simulink model "CryoDetHcd"  (R2016b)
settings: Solver=ode45  StartTime=0.0  StopTime=1e-3  RelTol=1e-3
PreLoadFcn:
  | setup_hcd
values from neighbouring files (symbols this model uses):
  A = sqrt(0.5*erfc(x))    [setup_hcd.m]
  Fadc = 307.2e6    (= 307200000)    [setupADCtoDACloopback.m]    (also in setupCryoFPGA_CMB.m; setup_hcd.m = 614000000)
undefined symbols (not defined in the file or in its folder): AXI4, B, C, D, etaRomData, freqRomData, freqRomData1, freqRomData2, freqRomData3, j, Lite
libraries: xbsIndex_r4 x897, CryoDetLibCMB x8, hdlsllib x8, dspsigops x2, simulink x1
(part 6 of 8)

== system CryoDetHcd/DspCore/DSP/analysis_pipelined/Analysis0/channel_select1 ==
  tready : Inport
  data_valid : Inport  Port=2
  Constant : xbsIndex_r4/Constant  const=6  gui_display_data_type=Fixed-point  arith_type=Unsigned  n_bits=3  bin_pt=0  preci_type=Single  exp_width=8  frac_width=24  explicit_period=off  period=1  equ=P=C  opselect=C  inp2=PCIN>>17  opr=+  inp1=P  carry=CIN  dbl_ovrd=off  block_type=constant
  Counter : xbsIndex_r4/Counter  cnt_type=Free Running  cnt_to=Inf  operation=Up  start_count=0  cnt_by_val=1  arith_type=Unsigned  n_bits=3  bin_pt=0  load_pin=off  rst=on  en=on  explicit_period=on  period=2/Fadc  use_behavioral_HDL=off  implementation=Fabric  dbl_ovrd=off  block_type=counter
  Logical6 : xbsIndex_r4/Logical  logical_function=AND  inputs=2  en=off  latency=1  precision=Full  arith_type=Unsigned  n_bits=16  bin_pt=0  align_bp=on  dbl_ovrd=off  block_type=logical
  Relational : xbsIndex_r4/Relational  mode=a=b  op_type=Bool  en=off  latency=1  dbl_ovrd=off  block_type=relational
  tvalid : Outport
  tdata_fsel : Outport  Port=2
  t_last : Outport  Port=3
  wires:
  Logical6/1 -> Counter/2, tvalid/1
  data_valid/1 -> Logical6/2
  Counter/1 -> Relational/2, tdata_fsel/1
  tready/1 -> Logical6/1
  Relational/1 -> t_last/1
  Constant/1 -> Relational/1
  [reset] -> Counter/1

== system CryoDetHcd/DspCore/DSP/analysis_pipelined/Analysis0/scale1 ==
  note: do we saturate here or later???
  sel : Inport
  valid_i : Inport  Port=2
  In1 : Inport  Port=3
  Convert2 : xbsIndex_r4/Convert  gui_display_data_type=Boolean  arith_type=Boolean  n_bits=16  bin_pt=15  float_type=Single  exp_bits=8  fraction_bits=24  quantization=Truncate  overflow=Flag as error  en=off  latency=0  pipeline=off  dbl_ovrd=off  block_type=convert
  Delay : xbsIndex_r4/Delay  rst=off  infoeditControl=Selection of Reset will increase slice count due to use of real FFs and instead of SRLs  en=off  latency=1  reg_retiming=off  dbl_ovrd=off  block_type=delay
  Delay1 : xbsIndex_r4/Delay  rst=off  infoeditControl=Selection of Reset will increase slice count due to use of real FFs and instead of SRLs  en=off  latency=1  reg_retiming=off  dbl_ovrd=off  block_type=delay
  Delay2 : xbsIndex_r4/Delay  rst=off  infoeditControl=Selection of Reset will increase slice count due to use of real FFs and instead of SRLs  en=off  latency=1  reg_retiming=off  dbl_ovrd=off  block_type=delay
  Mux1 : xbsIndex_r4/Mux  inputs=2  en=off  latency=1  precision=User Defined  arith_type="Signed  (2's comp)"  n_bits=18  bin_pt=17  quantization=Truncate  overflow=Saturate  dbl_ovrd=off  block_type=mux
  Mux2 : xbsIndex_r4/Mux  inputs=2  en=off  latency=1  precision=User Defined  arith_type="Signed  (2's comp)"  n_bits=18  bin_pt=17  quantization=Truncate  overflow=Saturate  dbl_ovrd=off  block_type=mux
  high : xbsIndex_r4/BitBasher  bitexpr=|  display_expr=off  sr_1=im_out  arith_type1="Signed  (2's comp)"  bin_pt1=17  sr_2=re_out  arith_type2="Signed  (2's comp)"  bin_pt2=17  sr_3=indx  arith_type3=Unsigned  bin_pt3=0  sr_4=tlast  arith_type4=Unsigned  bin_pt4=0  dbl_ovrd=off  block_type=bitbasher
      | im_out ={ in[39:21] }
      | re_out = { in[18:0] }
      | indx    = { in[44:42] } 
      | tlast     = { in[45] }
  slice8 : xbsIndex_r4/BitBasher  bitexpr=|  display_expr=off  sr_1=im_out  arith_type1="Signed  (2's comp)"  bin_pt1=17  sr_2=re_out  arith_type2="Signed  (2's comp)"  bin_pt2=17  sr_3=indx  arith_type3=Unsigned  bin_pt3=0  sr_4=tlast  arith_type4=Unsigned  bin_pt4=0  dbl_ovrd=off  block_type=bitbasher
      | im_out ={ in[39:22] }
      | re_out = { in[18:1] }
      | indx    = { in[44:42] } 
      | tlast     = { in[45] }
  valid_o : Outport
  im : Outport  Port=2
  re : Outport  Port=3
  indx : Outport  Port=4
  tlast : Outport  Port=5
  wires:
  Convert2/1 -> Delay2/1
  In1/1 -> slice8/1, high/1
  high/3 -> Delay1/1
  high/4 -> Convert2/1
  high/2 -> Mux1/3
  slice8/2 -> Mux1/2
  Mux1/1 -> re/1
  high/1 -> Mux2/3
  Delay2/1 -> tlast/1
  valid_i/1 -> Delay/1
  slice8/1 -> Mux2/2
  Delay/1 -> valid_o/1
  Mux2/1 -> im/1
  Delay1/1 -> indx/1
  sel/1 -> Mux2/1, Mux1/1

== system CryoDetHcd/DspCore/DSP/analysis_pipelined/Analysis0/scale2 ==
  note: do we saturate here or later???
  sel : Inport
  valid_i : Inport  Port=2
  In1 : Inport  Port=3
  Delay : xbsIndex_r4/Delay  rst=off  infoeditControl=Selection of Reset will increase slice count due to use of real FFs and instead of SRLs  en=off  latency=1  reg_retiming=off  dbl_ovrd=off  block_type=delay
  Delay1 : xbsIndex_r4/Delay  rst=off  infoeditControl=Selection of Reset will increase slice count due to use of real FFs and instead of SRLs  en=off  latency=1  reg_retiming=off  dbl_ovrd=off  block_type=delay
  Mux1 : xbsIndex_r4/Mux  inputs=2  en=off  latency=1  precision=User Defined  arith_type="Signed  (2's comp)"  n_bits=18  bin_pt=17  quantization=Truncate  overflow=Saturate  dbl_ovrd=off  block_type=mux
  Mux2 : xbsIndex_r4/Mux  inputs=2  en=off  latency=1  precision=User Defined  arith_type="Signed  (2's comp)"  n_bits=18  bin_pt=17  quantization=Truncate  overflow=Saturate  dbl_ovrd=off  block_type=mux
  high : xbsIndex_r4/BitBasher  bitexpr=|  display_expr=off  sr_1=re  arith_type1="Signed  (2's comp)"  bin_pt1=17  sr_2=im  arith_type2="Signed  (2's comp)"  bin_pt2=17  sr_3=indx  arith_type3=Unsigned  bin_pt3=0  sr_4=4  arith_type4=Unsigned  bin_pt4=0  dbl_ovrd=off  block_type=bitbasher
      | re={in[18:0]}
      | im={in[44:26]}
      | indx ={in[54:52]}
  nominal : xbsIndex_r4/BitBasher  bitexpr=|  display_expr=off  sr_1=re  arith_type1="Signed  (2's comp)"  bin_pt1=17  sr_2=im  arith_type2="Signed  (2's comp)"  bin_pt2=17  sr_3=indx  arith_type3=Unsigned  bin_pt3=0  sr_4=4  arith_type4=Unsigned  bin_pt4=0  dbl_ovrd=off  block_type=bitbasher
      | re={in[18:1]}
      | im={in[44:27]}
      | indx ={in[54:52]}
  valid_o : Outport
  re : Outport  Port=2
  im : Outport  Port=3
  indx : Outport  Port=4
  wires:
  sel/1 -> Mux1/1, Mux2/1
  Delay1/1 -> indx/1
  Delay/1 -> valid_o/1
  valid_i/1 -> Delay/1
  In1/1 -> nominal/1, high/1
  Mux2/1 -> re/1
  Mux1/1 -> im/1
  high/3 -> Delay1/1
  high/2 -> Mux1/3
  high/1 -> Mux2/3
  nominal/1 -> Mux2/2
  nominal/2 -> Mux1/2

== system CryoDetHcd/DspCore/DSP/analysis_pipelined/Analysis0/scale3 ==
  note: do we saturate here or later???
  sel : Inport
  valid_i : Inport  Port=2
  In1 : Inport  Port=3
  Delay : xbsIndex_r4/Delay  rst=off  infoeditControl=Selection of Reset will increase slice count due to use of real FFs and instead of SRLs  en=off  latency=1  reg_retiming=off  dbl_ovrd=off  block_type=delay
  Delay1 : xbsIndex_r4/Delay  rst=off  infoeditControl=Selection of Reset will increase slice count due to use of real FFs and instead of SRLs  en=off  latency=1  reg_retiming=off  dbl_ovrd=off  block_type=delay
  Mux1 : xbsIndex_r4/Mux  inputs=2  en=off  latency=1  precision=User Defined  arith_type="Signed  (2's comp)"  n_bits=18  bin_pt=17  quantization=Truncate  overflow=Saturate  dbl_ovrd=off  block_type=mux
  Mux2 : xbsIndex_r4/Mux  inputs=2  en=off  latency=1  precision=User Defined  arith_type="Signed  (2's comp)"  n_bits=18  bin_pt=17  quantization=Truncate  overflow=Saturate  dbl_ovrd=off  block_type=mux
  high : xbsIndex_r4/BitBasher  bitexpr=|  display_expr=off  sr_1=re  arith_type1="Signed  (2's comp)"  bin_pt1=17  sr_2=im  arith_type2="Signed  (2's comp)"  bin_pt2=17  sr_3=indx  arith_type3=Unsigned  bin_pt3=0  sr_4=4  arith_type4=Unsigned  bin_pt4=0  dbl_ovrd=off  block_type=bitbasher
      | re={in[18:0]}
      | im={in[44:26]}
      | indx ={in[54:52]}
  nominal : xbsIndex_r4/BitBasher  bitexpr=|  display_expr=off  sr_1=re  arith_type1="Signed  (2's comp)"  bin_pt1=17  sr_2=im  arith_type2="Signed  (2's comp)"  bin_pt2=17  sr_3=indx  arith_type3=Unsigned  bin_pt3=0  sr_4=4  arith_type4=Unsigned  bin_pt4=0  dbl_ovrd=off  block_type=bitbasher
      | re={in[18:1]}
      | im={in[44:27]}
      | indx ={in[54:52]}
  valid_o : Outport
  re : Outport  Port=2
  im : Outport  Port=3
  indx : Outport  Port=4
  wires:
  nominal/2 -> Mux1/2
  nominal/1 -> Mux2/2
  high/1 -> Mux2/3
  high/2 -> Mux1/3
  high/3 -> Delay1/1
  Mux1/1 -> im/1
  Mux2/1 -> re/1
  In1/1 -> high/1, nominal/1
  valid_i/1 -> Delay/1
  Delay/1 -> valid_o/1
  Delay1/1 -> indx/1
  sel/1 -> Mux2/1, Mux1/1

== system CryoDetHcd/DspCore/DSP/analysis_pipelined/Analysis0/scale4 ==
  note: do we saturate here or later???
  sel : Inport
  valid_i : Inport  Port=2
  In1 : Inport  Port=3
  Convert2 : xbsIndex_r4/Convert  gui_display_data_type=Boolean  arith_type=Boolean  n_bits=16  bin_pt=15  float_type=Single  exp_bits=8  fraction_bits=24  quantization=Truncate  overflow=Flag as error  en=off  latency=0  pipeline=off  dbl_ovrd=off  block_type=convert
  Delay : xbsIndex_r4/Delay  rst=off  infoeditControl=Selection of Reset will increase slice count due to use of real FFs and instead of SRLs  en=off  latency=1  reg_retiming=off  dbl_ovrd=off  block_type=delay
  Delay1 : xbsIndex_r4/Delay  rst=off  infoeditControl=Selection of Reset will increase slice count due to use of real FFs and instead of SRLs  en=off  latency=1  reg_retiming=off  dbl_ovrd=off  block_type=delay
  Delay2 : xbsIndex_r4/Delay  rst=off  infoeditControl=Selection of Reset will increase slice count due to use of real FFs and instead of SRLs  en=off  latency=1  reg_retiming=off  dbl_ovrd=off  block_type=delay
  Mux1 : xbsIndex_r4/Mux  inputs=2  en=off  latency=1  precision=User Defined  arith_type="Signed  (2's comp)"  n_bits=18  bin_pt=17  quantization=Truncate  overflow=Saturate  dbl_ovrd=off  block_type=mux
  Mux2 : xbsIndex_r4/Mux  inputs=2  en=off  latency=1  precision=User Defined  arith_type="Signed  (2's comp)"  n_bits=18  bin_pt=17  quantization=Truncate  overflow=Saturate  dbl_ovrd=off  block_type=mux
  high : xbsIndex_r4/BitBasher  bitexpr=|  display_expr=off  sr_1=im_out  arith_type1="Signed  (2's comp)"  bin_pt1=17  sr_2=re_out  arith_type2="Signed  (2's comp)"  bin_pt2=17  sr_3=indx  arith_type3=Unsigned  bin_pt3=0  sr_4=tlast  arith_type4=Unsigned  bin_pt4=0  dbl_ovrd=off  block_type=bitbasher
      | im_out ={ in[39:21] }
      | re_out = { in[18:0] }
      | indx    = { in[44:42] } 
      | tlast     = { in[45] }
  slice8 : xbsIndex_r4/BitBasher  bitexpr=|  display_expr=off  sr_1=im_out  arith_type1="Signed  (2's comp)"  bin_pt1=17  sr_2=re_out  arith_type2="Signed  (2's comp)"  bin_pt2=17  sr_3=indx  arith_type3=Unsigned  bin_pt3=0  sr_4=tlast  arith_type4=Unsigned  bin_pt4=0  dbl_ovrd=off  block_type=bitbasher
      | im_out ={ in[39:22] }
      | re_out = { in[18:1] }
      | indx    = { in[44:42] } 
      | tlast     = { in[45] }
  valid_o : Outport
  im : Outport  Port=2
  re : Outport  Port=3
  indx : Outport  Port=4
  tlast : Outport  Port=5
  wires:
  sel/1 -> Mux1/1, Mux2/1
  Delay1/1 -> indx/1
  Mux2/1 -> im/1
  Delay/1 -> valid_o/1
  slice8/1 -> Mux2/2
  valid_i/1 -> Delay/1
  Delay2/1 -> tlast/1
  high/1 -> Mux2/3
  Mux1/1 -> re/1
  slice8/2 -> Mux1/2
  high/2 -> Mux1/3
  high/4 -> Convert2/1
  high/3 -> Delay1/1
  In1/1 -> high/1, slice8/1
  Convert2/1 -> Delay2/1

== system CryoDetHcd/DspCore/DSP/analysis_pipelined/Analysis1/channel_select1 ==
  tready : Inport
  data_valid : Inport  Port=2
  Constant : xbsIndex_r4/Constant  const=6  gui_display_data_type=Fixed-point  arith_type=Unsigned  n_bits=3  bin_pt=0  preci_type=Single  exp_width=8  frac_width=24  explicit_period=off  period=1  equ=P=C  opselect=C  inp2=PCIN>>17  opr=+  inp1=P  carry=CIN  dbl_ovrd=off  block_type=constant
  Counter : xbsIndex_r4/Counter  cnt_type=Free Running  cnt_to=Inf  operation=Up  start_count=0  cnt_by_val=1  arith_type=Unsigned  n_bits=3  bin_pt=0  load_pin=off  rst=on  en=on  explicit_period=on  period=2/Fadc  use_behavioral_HDL=off  implementation=Fabric  dbl_ovrd=off  block_type=counter
  Logical6 : xbsIndex_r4/Logical  logical_function=AND  inputs=2  en=off  latency=1  precision=Full  arith_type=Unsigned  n_bits=16  bin_pt=0  align_bp=on  dbl_ovrd=off  block_type=logical
  Relational : xbsIndex_r4/Relational  mode=a=b  op_type=Bool  en=off  latency=1  dbl_ovrd=off  block_type=relational
  tvalid : Outport
  tdata_fsel : Outport  Port=2
  t_last : Outport  Port=3
  wires:
  [reset] -> Counter/1
  Constant/1 -> Relational/1
  Relational/1 -> t_last/1
  tready/1 -> Logical6/1
  Counter/1 -> tdata_fsel/1, Relational/2
  data_valid/1 -> Logical6/2
  Logical6/1 -> tvalid/1, Counter/2

== system CryoDetHcd/DspCore/DSP/analysis_pipelined/Analysis1/scale1 ==
  note: do we saturate here or later???
  sel : Inport
  valid_i : Inport  Port=2
  In1 : Inport  Port=3
  Convert2 : xbsIndex_r4/Convert  gui_display_data_type=Boolean  arith_type=Boolean  n_bits=16  bin_pt=15  float_type=Single  exp_bits=8  fraction_bits=24  quantization=Truncate  overflow=Flag as error  en=off  latency=0  pipeline=off  dbl_ovrd=off  block_type=convert
  Delay : xbsIndex_r4/Delay  rst=off  infoeditControl=Selection of Reset will increase slice count due to use of real FFs and instead of SRLs  en=off  latency=1  reg_retiming=off  dbl_ovrd=off  block_type=delay
  Delay1 : xbsIndex_r4/Delay  rst=off  infoeditControl=Selection of Reset will increase slice count due to use of real FFs and instead of SRLs  en=off  latency=1  reg_retiming=off  dbl_ovrd=off  block_type=delay
  Delay2 : xbsIndex_r4/Delay  rst=off  infoeditControl=Selection of Reset will increase slice count due to use of real FFs and instead of SRLs  en=off  latency=1  reg_retiming=off  dbl_ovrd=off  block_type=delay
  Mux1 : xbsIndex_r4/Mux  inputs=2  en=off  latency=1  precision=User Defined  arith_type="Signed  (2's comp)"  n_bits=18  bin_pt=17  quantization=Truncate  overflow=Saturate  dbl_ovrd=off  block_type=mux
  Mux2 : xbsIndex_r4/Mux  inputs=2  en=off  latency=1  precision=User Defined  arith_type="Signed  (2's comp)"  n_bits=18  bin_pt=17  quantization=Truncate  overflow=Saturate  dbl_ovrd=off  block_type=mux
  high : xbsIndex_r4/BitBasher  bitexpr=|  display_expr=off  sr_1=im_out  arith_type1="Signed  (2's comp)"  bin_pt1=17  sr_2=re_out  arith_type2="Signed  (2's comp)"  bin_pt2=17  sr_3=indx  arith_type3=Unsigned  bin_pt3=0  sr_4=tlast  arith_type4=Unsigned  bin_pt4=0  dbl_ovrd=off  block_type=bitbasher
      | im_out ={ in[39:21] }
      | re_out = { in[18:0] }
      | indx    = { in[44:42] } 
      | tlast     = { in[45] }
  slice8 : xbsIndex_r4/BitBasher  bitexpr=|  display_expr=off  sr_1=im_out  arith_type1="Signed  (2's comp)"  bin_pt1=17  sr_2=re_out  arith_type2="Signed  (2's comp)"  bin_pt2=17  sr_3=indx  arith_type3=Unsigned  bin_pt3=0  sr_4=tlast  arith_type4=Unsigned  bin_pt4=0  dbl_ovrd=off  block_type=bitbasher
      | im_out ={ in[39:22] }
      | re_out = { in[18:1] }
      | indx    = { in[44:42] } 
      | tlast     = { in[45] }
  valid_o : Outport
  im : Outport  Port=2
  re : Outport  Port=3
  indx : Outport  Port=4
  tlast : Outport  Port=5
  wires:
  sel/1 -> Mux1/1, Mux2/1
  Delay1/1 -> indx/1
  Mux2/1 -> im/1
  Delay/1 -> valid_o/1
  slice8/1 -> Mux2/2
  valid_i/1 -> Delay/1
  Delay2/1 -> tlast/1
  high/1 -> Mux2/3
  Mux1/1 -> re/1
  slice8/2 -> Mux1/2
  high/2 -> Mux1/3
  high/4 -> Convert2/1
  high/3 -> Delay1/1
  In1/1 -> high/1, slice8/1
  Convert2/1 -> Delay2/1

== system CryoDetHcd/DspCore/DSP/analysis_pipelined/Analysis1/scale2 ==
  note: do we saturate here or later???
  sel : Inport
  valid_i : Inport  Port=2
  In1 : Inport  Port=3
  Delay : xbsIndex_r4/Delay  rst=off  infoeditControl=Selection of Reset will increase slice count due to use of real FFs and instead of SRLs  en=off  latency=1  reg_retiming=off  dbl_ovrd=off  block_type=delay
  Delay1 : xbsIndex_r4/Delay  rst=off  infoeditControl=Selection of Reset will increase slice count due to use of real FFs and instead of SRLs  en=off  latency=1  reg_retiming=off  dbl_ovrd=off  block_type=delay
  Mux1 : xbsIndex_r4/Mux  inputs=2  en=off  latency=1  precision=User Defined  arith_type="Signed  (2's comp)"  n_bits=18  bin_pt=17  quantization=Truncate  overflow=Saturate  dbl_ovrd=off  block_type=mux
  Mux2 : xbsIndex_r4/Mux  inputs=2  en=off  latency=1  precision=User Defined  arith_type="Signed  (2's comp)"  n_bits=18  bin_pt=17  quantization=Truncate  overflow=Saturate  dbl_ovrd=off  block_type=mux
  high : xbsIndex_r4/BitBasher  bitexpr=|  display_expr=off  sr_1=re  arith_type1="Signed  (2's comp)"  bin_pt1=17  sr_2=im  arith_type2="Signed  (2's comp)"  bin_pt2=17  sr_3=indx  arith_type3=Unsigned  bin_pt3=0  sr_4=4  arith_type4=Unsigned  bin_pt4=0  dbl_ovrd=off  block_type=bitbasher
      | re={in[18:0]}
      | im={in[44:26]}
      | indx ={in[54:52]}
  nominal : xbsIndex_r4/BitBasher  bitexpr=|  display_expr=off  sr_1=re  arith_type1="Signed  (2's comp)"  bin_pt1=17  sr_2=im  arith_type2="Signed  (2's comp)"  bin_pt2=17  sr_3=indx  arith_type3=Unsigned  bin_pt3=0  sr_4=4  arith_type4=Unsigned  bin_pt4=0  dbl_ovrd=off  block_type=bitbasher
      | re={in[18:1]}
      | im={in[44:27]}
      | indx ={in[54:52]}
  valid_o : Outport
  re : Outport  Port=2
  im : Outport  Port=3
  indx : Outport  Port=4
  wires:
  nominal/2 -> Mux1/2
  nominal/1 -> Mux2/2
  high/1 -> Mux2/3
  high/2 -> Mux1/3
  high/3 -> Delay1/1
  Mux1/1 -> im/1
  Mux2/1 -> re/1
  In1/1 -> high/1, nominal/1
  valid_i/1 -> Delay/1
  Delay/1 -> valid_o/1
  Delay1/1 -> indx/1
  sel/1 -> Mux2/1, Mux1/1

== system CryoDetHcd/DspCore/DSP/analysis_pipelined/Analysis1/scale3 ==
  note: do we saturate here or later???
  sel : Inport
  valid_i : Inport  Port=2
  In1 : Inport  Port=3
  Delay : xbsIndex_r4/Delay  rst=off  infoeditControl=Selection of Reset will increase slice count due to use of real FFs and instead of SRLs  en=off  latency=1  reg_retiming=off  dbl_ovrd=off  block_type=delay
  Delay1 : xbsIndex_r4/Delay  rst=off  infoeditControl=Selection of Reset will increase slice count due to use of real FFs and instead of SRLs  en=off  latency=1  reg_retiming=off  dbl_ovrd=off  block_type=delay
  Mux1 : xbsIndex_r4/Mux  inputs=2  en=off  latency=1  precision=User Defined  arith_type="Signed  (2's comp)"  n_bits=18  bin_pt=17  quantization=Truncate  overflow=Saturate  dbl_ovrd=off  block_type=mux
  Mux2 : xbsIndex_r4/Mux  inputs=2  en=off  latency=1  precision=User Defined  arith_type="Signed  (2's comp)"  n_bits=18  bin_pt=17  quantization=Truncate  overflow=Saturate  dbl_ovrd=off  block_type=mux
  high : xbsIndex_r4/BitBasher  bitexpr=|  display_expr=off  sr_1=re  arith_type1="Signed  (2's comp)"  bin_pt1=17  sr_2=im  arith_type2="Signed  (2's comp)"  bin_pt2=17  sr_3=indx  arith_type3=Unsigned  bin_pt3=0  sr_4=4  arith_type4=Unsigned  bin_pt4=0  dbl_ovrd=off  block_type=bitbasher
      | re={in[18:0]}
      | im={in[44:26]}
      | indx ={in[54:52]}
  nominal : xbsIndex_r4/BitBasher  bitexpr=|  display_expr=off  sr_1=re  arith_type1="Signed  (2's comp)"  bin_pt1=17  sr_2=im  arith_type2="Signed  (2's comp)"  bin_pt2=17  sr_3=indx  arith_type3=Unsigned  bin_pt3=0  sr_4=4  arith_type4=Unsigned  bin_pt4=0  dbl_ovrd=off  block_type=bitbasher
      | re={in[18:1]}
      | im={in[44:27]}
      | indx ={in[54:52]}
  valid_o : Outport
  re : Outport  Port=2
  im : Outport  Port=3
  indx : Outport  Port=4
  wires:
  sel/1 -> Mux1/1, Mux2/1
  Delay1/1 -> indx/1
  Delay/1 -> valid_o/1
  valid_i/1 -> Delay/1
  In1/1 -> nominal/1, high/1
  Mux2/1 -> re/1
  Mux1/1 -> im/1
  high/3 -> Delay1/1
  high/2 -> Mux1/3
  high/1 -> Mux2/3
  nominal/1 -> Mux2/2
  nominal/2 -> Mux1/2

== system CryoDetHcd/DspCore/DSP/analysis_pipelined/Analysis1/scale4 ==
  note: do we saturate here or later???
  sel : Inport
  valid_i : Inport  Port=2
  In1 : Inport  Port=3
  Convert2 : xbsIndex_r4/Convert  gui_display_data_type=Boolean  arith_type=Boolean  n_bits=16  bin_pt=15  float_type=Single  exp_bits=8  fraction_bits=24  quantization=Truncate  overflow=Flag as error  en=off  latency=0  pipeline=off  dbl_ovrd=off  block_type=convert
  Delay : xbsIndex_r4/Delay  rst=off  infoeditControl=Selection of Reset will increase slice count due to use of real FFs and instead of SRLs  en=off  latency=1  reg_retiming=off  dbl_ovrd=off  block_type=delay
  Delay1 : xbsIndex_r4/Delay  rst=off  infoeditControl=Selection of Reset will increase slice count due to use of real FFs and instead of SRLs  en=off  latency=1  reg_retiming=off  dbl_ovrd=off  block_type=delay
  Delay2 : xbsIndex_r4/Delay  rst=off  infoeditControl=Selection of Reset will increase slice count due to use of real FFs and instead of SRLs  en=off  latency=1  reg_retiming=off  dbl_ovrd=off  block_type=delay
  Mux1 : xbsIndex_r4/Mux  inputs=2  en=off  latency=1  precision=User Defined  arith_type="Signed  (2's comp)"  n_bits=18  bin_pt=17  quantization=Truncate  overflow=Saturate  dbl_ovrd=off  block_type=mux
  Mux2 : xbsIndex_r4/Mux  inputs=2  en=off  latency=1  precision=User Defined  arith_type="Signed  (2's comp)"  n_bits=18  bin_pt=17  quantization=Truncate  overflow=Saturate  dbl_ovrd=off  block_type=mux
  high : xbsIndex_r4/BitBasher  bitexpr=|  display_expr=off  sr_1=im_out  arith_type1="Signed  (2's comp)"  bin_pt1=17  sr_2=re_out  arith_type2="Signed  (2's comp)"  bin_pt2=17  sr_3=indx  arith_type3=Unsigned  bin_pt3=0  sr_4=tlast  arith_type4=Unsigned  bin_pt4=0  dbl_ovrd=off  block_type=bitbasher
      | im_out ={ in[39:21] }
      | re_out = { in[18:0] }
      | indx    = { in[44:42] } 
      | tlast     = { in[45] }
  slice8 : xbsIndex_r4/BitBasher  bitexpr=|  display_expr=off  sr_1=im_out  arith_type1="Signed  (2's comp)"  bin_pt1=17  sr_2=re_out  arith_type2="Signed  (2's comp)"  bin_pt2=17  sr_3=indx  arith_type3=Unsigned  bin_pt3=0  sr_4=tlast  arith_type4=Unsigned  bin_pt4=0  dbl_ovrd=off  block_type=bitbasher
      | im_out ={ in[39:22] }
      | re_out = { in[18:1] }
      | indx    = { in[44:42] } 
      | tlast     = { in[45] }
  valid_o : Outport
  im : Outport  Port=2
  re : Outport  Port=3
  indx : Outport  Port=4
  tlast : Outport  Port=5
  wires:
  Convert2/1 -> Delay2/1
  In1/1 -> slice8/1, high/1
  high/3 -> Delay1/1
  high/4 -> Convert2/1
  high/2 -> Mux1/3
  slice8/2 -> Mux1/2
  Mux1/1 -> re/1
  high/1 -> Mux2/3
  Delay2/1 -> tlast/1
  valid_i/1 -> Delay/1
  slice8/1 -> Mux2/2
  Delay/1 -> valid_o/1
  Mux2/1 -> im/1
  Delay1/1 -> indx/1
  sel/1 -> Mux2/1, Mux1/1

== system CryoDetHcd/DspCore/DSP/channel_processor/channel_processor_x1/Enabled Subsystem ==
  In1 : Inport
  In2 : Inport  Port=2
  Enable : EnablePort
  Buffer : Buffer  N=8  TreatMby1Signals=One channel  OutputFrames=off
  Buffer1 : Buffer  N=8  TreatMby1Signals=One channel  OutputFrames=off
  Out1 : Outport
  Out2 : Outport  Port=2
  wires:
  In1/1 -> Buffer/1
  Buffer/1 -> Out1/1
  In2/1 -> Buffer1/1
  Buffer1/1 -> Out2/1

== system CryoDetHcd/DspCore/DSP/channel_processor/channel_processor_x1/IQ_status_sel ==
  sel : Inport
  Q : Inport  Port=2
  I : Inport  Port=3
  ch : Inport  Port=4
  BitBasher : xbsIndex_r4/BitBasher  bitexpr=out = {I,Q}  display_expr=off  sr_1=out  arith_type1=Unsigned  bin_pt1=0  sr_2=2  arith_type2=Unsigned  bin_pt2=0  sr_3=3  arith_type3=Unsigned  bin_pt3=0  sr_4=4  arith_type4=Unsigned  bin_pt4=0  dbl_ovrd=off  block_type=bitbasher
  Convert : xbsIndex_r4/Convert  gui_display_data_type=Fixed-point  arith_type="Signed  (2's comp)"  n_bits=16  bin_pt=15  float_type=Single  exp_bits=8  fraction_bits=24  quantization=Truncate  overflow=Wrap  en=off  latency=1  pipeline=off  dbl_ovrd=off  block_type=convert
  Convert1 : xbsIndex_r4/Convert  gui_display_data_type=Fixed-point  arith_type="Signed  (2's comp)"  n_bits=16  bin_pt=15  float_type=Single  exp_bits=8  fraction_bits=24  quantization=Truncate  overflow=Wrap  en=off  latency=1  pipeline=off  dbl_ovrd=off  block_type=convert
  Register2 : xbsIndex_r4/Register  init=0  rst=off  en=on  dbl_ovrd=off  block_type=register
  Relational : xbsIndex_r4/Relational  mode=a=b  op_type=Bool  en=off  latency=1  dbl_ovrd=off  block_type=relational
  IQ_status_r : Outport
  wires:
  I/1 -> Convert1/1
  Q/1 -> Convert/1
  Convert1/1 -> BitBasher/2
  ch/1 -> Relational/2
  sel/1 -> Relational/1
  Convert/1 -> BitBasher/1
  BitBasher/1 -> Register2/1
  Register2/1 -> IQ_status_r/1
  Relational/1 -> Register2/2

== system CryoDetHcd/DspCore/DSP/channel_processor/channel_processor_x1/config2_r ==
  In1 : Inport
  BitBasher : xbsIndex_r4/BitBasher  bitexpr=|  display_expr=off  sr_1=ref_delay  arith_type1=Unsigned  bin_pt1=0  sr_2=tone_scale_sel  arith_type2=Unsigned  bin_pt2=0  sr_3=fb_enable  arith_type3=Unsigned  bin_pt3=0  sr_4=fb_polarity  arith_type4=Unsigned  bin_pt4=0  dbl_ovrd=off  block_type=bitbasher
      | ref_delay = {in[2:0]}
      | tone_scale_sel = {in[4:3]}
      | fb_enable = {in[5]}
      | fb_polarity = {in[6]}
  BitBasher1 : xbsIndex_r4/BitBasher  bitexpr=|  display_expr=off  sr_1=iq_swap_sel  arith_type1=Unsigned  bin_pt1=0  sr_2=iq_band_sel  arith_type2=Unsigned  bin_pt2=0  sr_3=iq_ch_sel  arith_type3=Unsigned  bin_pt3=0  sr_4=analysis_iq_ch_sel  arith_type4=Unsigned  bin_pt4=0  dbl_ovrd=off  block_type=bitbasher
      | iq_swap_sel = {in[7]}
      | iq_band_sel = {in[16:15]}
      | iq_ch_sel = {in[14:8]}
      | analysis_iq_ch_sel={in[17:15]}
  ref_delay : Outport
  tone_scale_sel : Outport  Port=2
  fb_enable : Outport  Port=3
  fb_polarity : Outport  Port=4
  iq_swap_sel : Outport  Port=5
  iq_band_sel : Outport  Port=6
  iq_ch_sel : Outport  Port=7
  analysis_iq_sel : Outport  Port=8
  wires:
  BitBasher1/3 -> iq_ch_sel/1
  BitBasher1/2 -> iq_band_sel/1
  BitBasher1/1 -> iq_swap_sel/1
  BitBasher/4 -> fb_polarity/1
  BitBasher/3 -> fb_enable/1
  BitBasher/2 -> tone_scale_sel/1
  BitBasher/1 -> ref_delay/1
  In1/1 -> BitBasher/1, BitBasher1/1
  BitBasher1/4 -> analysis_iq_sel/1

== system CryoDetHcd/DspCore/DSP/channel_processor/channel_processor_x1/config3_r1 ==
  In1 : Inport
  BitBasher1 : xbsIndex_r4/BitBasher  bitexpr=|  display_expr=off  sr_1=fb_gain  arith_type1=Unsigned  bin_pt1=14  sr_2=fb_limit  arith_type2=Unsigned  bin_pt2=16  sr_3=ref_delay  arith_type3=Unsigned  bin_pt3=0  sr_4=4  arith_type4=Unsigned  bin_pt4=0  dbl_ovrd=off  block_type=bitbasher
      | fb_gain = {in[15:0]}
      | fb_limit = {in[31:16]}
  Negate : xbsIndex_r4/Negate  precision=User Defined  arith_type=Unsigned  n_bits=16  bin_pt=15  quantization=Truncate  overflow=Wrap  en=off  latency=2  dbl_ovrd=off  block_type=negate
  fb_gain : Outport
  fb_limit_hi : Outport  Port=2
  fb_limit_lo : Outport  Port=3
  wires:
  BitBasher1/2 -> Negate/1, fb_limit_hi/1
  In1/1 -> BitBasher1/1
  BitBasher1/1 -> fb_gain/1
  Negate/1 -> fb_limit_lo/1

== system CryoDetHcd/DspCore/DSP/channel_processor/channel_processor_x1/scale1 ==
  In1 : Inport
  Bit Slice : hdlsllib/HDL Operations/Bit Slice  lidx=15  ridx=0
  Bit Slice1 : hdlsllib/HDL Operations/Bit Slice  lidx=31  ridx=16
  Data Type Conversion : DataTypeConversion  OutDataTypeStr=int16  ConvertRealWorld=Stored Integer (SI)
  Data Type Conversion1 : DataTypeConversion  OutDataTypeStr=int16  ConvertRealWorld=Stored Integer (SI)
  Q : Outport
  I : Outport  Port=2
  wires:
  In1/1 -> Bit Slice1/1, Bit Slice/1
  Bit Slice/1 -> Data Type Conversion/1
  Data Type Conversion1/1 -> Q/1
  Bit Slice1/1 -> Data Type Conversion1/1
  Data Type Conversion/1 -> I/1

== system CryoDetHcd/DspCore/DSP/channel_processor/channel_processor_x4/Enabled Subsystem ==
  In1 : Inport
  In2 : Inport  Port=2
  Enable : EnablePort
  Buffer : Buffer  N=8  TreatMby1Signals=One channel  OutputFrames=off
  Buffer1 : Buffer  N=8  TreatMby1Signals=One channel  OutputFrames=off
  Out1 : Outport
  Out2 : Outport  Port=2
  wires:
  In1/1 -> Buffer/1
  Buffer/1 -> Out1/1
  In2/1 -> Buffer1/1
  Buffer1/1 -> Out2/1

== system CryoDetHcd/DspCore/DSP/channel_processor/channel_processor_x4/config3_r ==
  In1 : Inport
  BitBasher1 : xbsIndex_r4/BitBasher  bitexpr=|  display_expr=off  sr_1=fb_gain  arith_type1=Unsigned  bin_pt1=14  sr_2=fb_limit  arith_type2=Unsigned  bin_pt2=16  sr_3=ref_delay  arith_type3=Unsigned  bin_pt3=0  sr_4=4  arith_type4=Unsigned  bin_pt4=0  dbl_ovrd=off  block_type=bitbasher
      | fb_gain = {in[15:0]}
      | fb_limit = {in[31:16]}
  Negate : xbsIndex_r4/Negate  precision=User Defined  arith_type=Unsigned  n_bits=16  bin_pt=15  quantization=Truncate  overflow=Wrap  en=off  latency=2  dbl_ovrd=off  block_type=negate
  fb_gain : Outport
  fb_limit_hi : Outport  Port=2
  fb_limit_lo : Outport  Port=3
  wires:
  BitBasher1/2 -> Negate/1, fb_limit_hi/1
  In1/1 -> BitBasher1/1
  BitBasher1/1 -> fb_gain/1
  Negate/1 -> fb_limit_lo/1

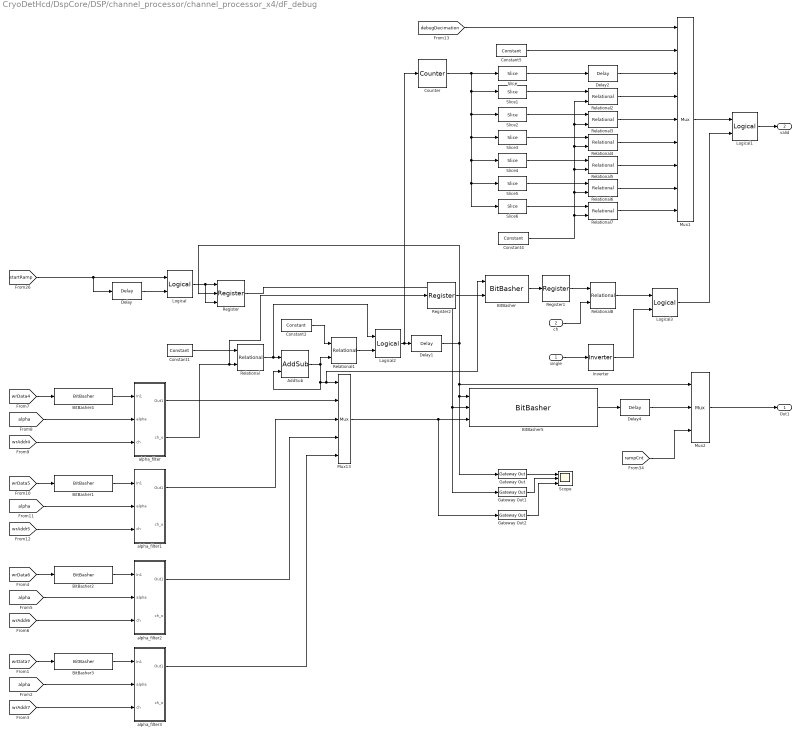
== system CryoDetHcd/DspCore/DSP/channel_processor/channel_processor_x4/dF_debug ==
  single : Inport
  ch : Inport  Port=2
  AddSub : xbsIndex_r4/AddSub  mode=Addition  use_carryin=off  use_carryout=off  en=off  latency=1  precision=User Defined  arith_type=Unsigned  n_bits=2  bin_pt=0  quantization=Truncate  overflow=Wrap  use_behavioral_HDL=off  hw_selection=Fabric  pipelined=off  dbl_ovrd=off  block_type=addsub
  BitBasher : xbsIndex_r4/BitBasher  bitexpr=out = {hi,lo}  display_expr=off  sr_1=out  arith_type1=Unsigned  bin_pt1=0  sr_2=channel_select  arith_type2=Unsigned  bin_pt2=0  sr_3=3  arith_type3=Unsigned  bin_pt3=0  sr_4=4  arith_type4=Unsigned  bin_pt4=0  dbl_ovrd=off  block_type=bitbasher
  BitBasher{1..4} (4 alike) : xbsIndex_r4/BitBasher  bitexpr=freq = {in[23:0]}  display_expr=on  sr_1=freq  arith_type1="Signed  (2's comp)"  bin_pt1=0  sr_2=2  arith_type2=Unsigned  bin_pt2=0  sr_3=3  arith_type3=Unsigned  bin_pt3=0  sr_4=4  arith_type4=Unsigned  bin_pt4=0  dbl_ovrd=off  block_type=bitbasher
  BitBasher5 : xbsIndex_r4/BitBasher  bitexpr=out = {flux_ramp, ch, 6'b0, freq}  display_expr=on  sr_1=out  arith_type1=Unsigned  bin_pt1=0  sr_2=2  arith_type2=Unsigned  bin_pt2=0  sr_3=3  arith_type3=Unsigned  bin_pt3=0  sr_4=4  arith_type4=Unsigned  bin_pt4=0  dbl_ovrd=off  block_type=bitbasher
  Constant1 : xbsIndex_r4/Constant  const=127  gui_display_data_type=Fixed-point  arith_type=Unsigned  n_bits=7  bin_pt=0  preci_type=Single  exp_width=8  frac_width=24  explicit_period=off  period=1  equ=P=C  opselect=C  inp2=PCIN>>17  opr=+  inp1=P  carry=CIN  dbl_ovrd=off  block_type=constant
  Constant2 : xbsIndex_r4/Constant  const=3  gui_display_data_type=Fixed-point  arith_type=Unsigned  n_bits=2  bin_pt=0  preci_type=Single  exp_width=8  frac_width=24  explicit_period=off  period=1  equ=P=C  opselect=C  inp2=PCIN>>17  opr=+  inp1=P  carry=CIN  dbl_ovrd=off  block_type=constant
  Constant4 : xbsIndex_r4/Constant  const=0  gui_display_data_type=Fixed-point  arith_type=Unsigned  n_bits=1  bin_pt=0  preci_type=Single  exp_width=8  frac_width=24  explicit_period=off  period=1  equ=P=C  opselect=C  inp2=PCIN>>17  opr=+  inp1=P  carry=CIN  dbl_ovrd=off  block_type=constant
  Constant5 : xbsIndex_r4/Constant  const=1  gui_display_data_type=Fixed-point  arith_type=Unsigned  n_bits=1  bin_pt=0  preci_type=Single  exp_width=8  frac_width=24  explicit_period=off  period=1  equ=P=C  opselect=C  inp2=PCIN>>17  opr=+  inp1=P  carry=CIN  dbl_ovrd=off  block_type=constant
  Counter : xbsIndex_r4/Counter  cnt_type=Free Running  cnt_to=Inf  operation=Up  start_count=0  cnt_by_val=1  arith_type=Unsigned  n_bits=7  bin_pt=0  load_pin=off  rst=off  en=on  explicit_period=off  period=2/Fadc  use_behavioral_HDL=off  implementation=Fabric  dbl_ovrd=off  block_type=counter
  Delay{,1..2,4} (4 alike) : xbsIndex_r4/Delay  rst=off  infoeditControl=Selection of Reset will increase slice count due to use of real FFs and instead of SRLs  en=off  latency=1  reg_retiming=off  dbl_ovrd=off  block_type=delay
  Gateway Out : xbsIndex_r4/Gateway Out  inherit_from_input=off  hdl_port=off  rows=1  columns=1  UseAsDAC=off  DACChannel='1'  interface=None  automatic_assignment=on  address_offset=hex2dec('00')  intf_name=''  intf_description=''  timing_constraint=None  locs_specified=off  LOCs={}  io_standard={}  block_type=gatewayout
  Gateway Out1 : xbsIndex_r4/Gateway Out  inherit_from_input=off  hdl_port=off  rows=1  columns=1  UseAsDAC=off  DACChannel='1'  interface=None  automatic_assignment=on  address_offset=hex2dec('00')  intf_name=''  intf_description=''  timing_constraint=None  locs_specified=off  LOCs={}  io_standard={}  block_type=gatewayout
  Gateway Out2 : xbsIndex_r4/Gateway Out  inherit_from_input=off  hdl_port=off  rows=1  columns=1  UseAsDAC=off  DACChannel='1'  interface=None  automatic_assignment=on  address_offset=hex2dec('00')  intf_name=''  intf_description=''  timing_constraint=None  locs_specified=off  LOCs={}  io_standard={}  block_type=gatewayout
  Inverter : xbsIndex_r4/Inverter  en=off  latency=0  dbl_ovrd=off  block_type=inv
  Logical : xbsIndex_r4/Logical  logical_function=OR  inputs=2  en=off  latency=1  precision=User Defined  arith_type=Boolean  n_bits=16  bin_pt=0  align_bp=on  dbl_ovrd=off  block_type=logical
  Logical1 : xbsIndex_r4/Logical  logical_function=AND  inputs=2  en=off  latency=0  precision=Full  arith_type=Unsigned  n_bits=16  bin_pt=0  align_bp=on  dbl_ovrd=off  block_type=logical
  Logical2 : xbsIndex_r4/Logical  logical_function=AND  inputs=2  en=off  latency=1  precision=User Defined  arith_type=Boolean  n_bits=16  bin_pt=0  align_bp=on  dbl_ovrd=off  block_type=logical
  Logical3 : xbsIndex_r4/Logical  logical_function=OR  inputs=2  en=off  latency=1  precision=Full  arith_type=Unsigned  n_bits=16  bin_pt=0  align_bp=on  dbl_ovrd=off  block_type=logical
  Mux1 : xbsIndex_r4/Mux  inputs=8  en=off  latency=1  precision=Full  arith_type=Unsigned  n_bits=16  bin_pt=14  quantization=Truncate  overflow=Wrap  dbl_ovrd=off  block_type=mux
  Mux13 : xbsIndex_r4/Mux  inputs=4  en=off  latency=1  precision=Full  arith_type=Unsigned  n_bits=16  bin_pt=14  quantization=Truncate  overflow=Wrap  dbl_ovrd=off  block_type=mux
  Mux2 : xbsIndex_r4/Mux  inputs=2  en=off  latency=1  precision=Full  arith_type=Unsigned  n_bits=16  bin_pt=14  quantization=Truncate  overflow=Wrap  dbl_ovrd=off  block_type=mux
  Register : xbsIndex_r4/Register  init=0  rst=on  en=on  dbl_ovrd=off  block_type=register
  Register1 : xbsIndex_r4/Register  init=0  rst=off  en=off  dbl_ovrd=off  block_type=register
  Register2 : xbsIndex_r4/Register  init=0  rst=off  en=off  dbl_ovrd=off  block_type=register
  Relational{,1..8} (9 alike) : xbsIndex_r4/Relational  mode=a=b  op_type=Ufix  en=off  latency=1  dbl_ovrd=off  block_type=relational
  Scope : Scope  NumInputPorts=3
  Slice : xbsIndex_r4/Slice  nbits=1  boolean_output=off  mode=Lower Bit Location + Width  bit1=0  base1=MSB of Input  bit0=0  base0=LSB of Input  dbl_ovrd=off  block_type=slice
  Slice1 : xbsIndex_r4/Slice  nbits=2  boolean_output=off  mode=Lower Bit Location + Width  bit1=0  base1=MSB of Input  bit0=0  base0=LSB of Input  dbl_ovrd=off  block_type=slice
  Slice2 : xbsIndex_r4/Slice  nbits=3  boolean_output=off  mode=Lower Bit Location + Width  bit1=0  base1=MSB of Input  bit0=0  base0=LSB of Input  dbl_ovrd=off  block_type=slice
  Slice3 : xbsIndex_r4/Slice  nbits=4  boolean_output=off  mode=Lower Bit Location + Width  bit1=0  base1=MSB of Input  bit0=0  base0=LSB of Input  dbl_ovrd=off  block_type=slice
  Slice4 : xbsIndex_r4/Slice  nbits=5  boolean_output=off  mode=Lower Bit Location + Width  bit1=0  base1=MSB of Input  bit0=0  base0=LSB of Input  dbl_ovrd=off  block_type=slice
  Slice5 : xbsIndex_r4/Slice  nbits=6  boolean_output=off  mode=Lower Bit Location + Width  bit1=0  base1=MSB of Input  bit0=0  base0=LSB of Input  dbl_ovrd=off  block_type=slice
  Slice6 : xbsIndex_r4/Slice  nbits=7  boolean_output=off  mode=Lower Bit Location + Width  bit1=0  base1=MSB of Input  bit0=0  base0=LSB of Input  dbl_ovrd=off  block_type=slice
  alpha_filter : Subsystem
  alpha_filter1 : Subsystem
  alpha_filter2 : Subsystem
  alpha_filter3 : Subsystem
  Out1 : Outport
  valid : Outport  Port=2
  wires:
  [wrData5] -> BitBasher1/1
  [alpha] -> alpha_filter1/2(alpha)
  [wrAddr4] -> alpha_filter/3(ch)
  [wrAddr5] -> alpha_filter1/3(ch)
  BitBasher1/1 -> alpha_filter1/1(In1)
  [alpha] -> alpha_filter/2(alpha)
  [wrData4] -> BitBasher4/1
  BitBasher4/1 -> alpha_filter/1(In1)
  [wrData7] -> BitBasher3/1
  [alpha] -> alpha_filter3/2(alpha)
  [wrAddr6] -> alpha_filter2/3(ch)
  [wrAddr7] -> alpha_filter3/3(ch)
  BitBasher3/1 -> alpha_filter3/1(In1)
  [alpha] -> alpha_filter2/2(alpha)
  [wrData6] -> BitBasher2/1
  BitBasher2/1 -> alpha_filter2/1(In1)
  alpha_filter/1(Out1) -> Mux13/2
  alpha_filter1/1(Out1) -> Mux13/3
  alpha_filter2/1(Out1) -> Mux13/4
  alpha_filter3/1(Out1) -> Mux13/5
  Delay/1 -> Logical/2
  [startRamp] -> Delay/1, Logical/1
  Logical/1 -> Register/3, Register/1
  alpha_filter/2(ch_o) -> Register2/1, Relational/2
  Constant1/1 -> Relational/1
  Constant2/1 -> Relational1/1
  Mux13/1 -> Gateway Out2/1, BitBasher5/3
  Relational1/1 -> Logical2/2
  Register/1 -> Gateway Out1/1, BitBasher5/2
  Relational/1 -> Logical2/1, AddSub/1
  Gateway Out/1 -> Scope/1
  Gateway Out1/1 -> Scope/2
  Gateway Out2/1 -> Scope/3
  Counter/1 -> Slice3/1, Slice4/1, Slice5/1, Slice6/1, Slice2/1, Slice1/1, Slice/1
  Logical2/1 -> Counter/1, Delay1/1
  Slice1/1 -> Relational2/1
  Slice2/1 -> Relational3/1
  Constant4/1 -> Relational2/2, Relational3/2, Relational4/2, Relational5/2, Relational6/2, Relational7/2
  Relational6/1 -> Mux1/8
  Relational5/1 -> Mux1/7
  Relational4/1 -> Mux1/6
  Relational3/1 -> Mux1/5
  Relational2/1 -> Mux1/4
  Delay2/1 -> Mux1/3
  Slice/1 -> Delay2/1
  Slice3/1 -> Relational4/1
  Slice4/1 -> Relational5/1
  Slice5/1 -> Relational6/1
  Slice6/1 -> Relational7/1
  Constant5/1 -> Mux1/2
  Relational7/1 -> Mux1/9
  Delay1/1 -> Register/2, Mux2/1, Gateway Out/1, BitBasher5/1
  Delay4/1 -> Mux2/2
  [rampCnt] -> Mux2/3
  BitBasher5/1 -> Delay4/1
  Mux2/1 -> Out1/1
  AddSub/1 -> AddSub/2, BitBasher/1, Mux13/1, Relational1/2
  BitBasher/1 -> Register1/1
  Register2/1 -> BitBasher/2
  Register1/1 -> Relational8/1
  Relational8/1 -> Logical3/1
  Logical3/1 -> Logical1/2
  ch/1 -> Relational8/2
  single/1 -> Inverter/1
  Inverter/1 -> Logical3/2
  Mux1/1 -> Logical1/1
  Logical1/1 -> valid/1
  [debugDecimation] -> Mux1/1

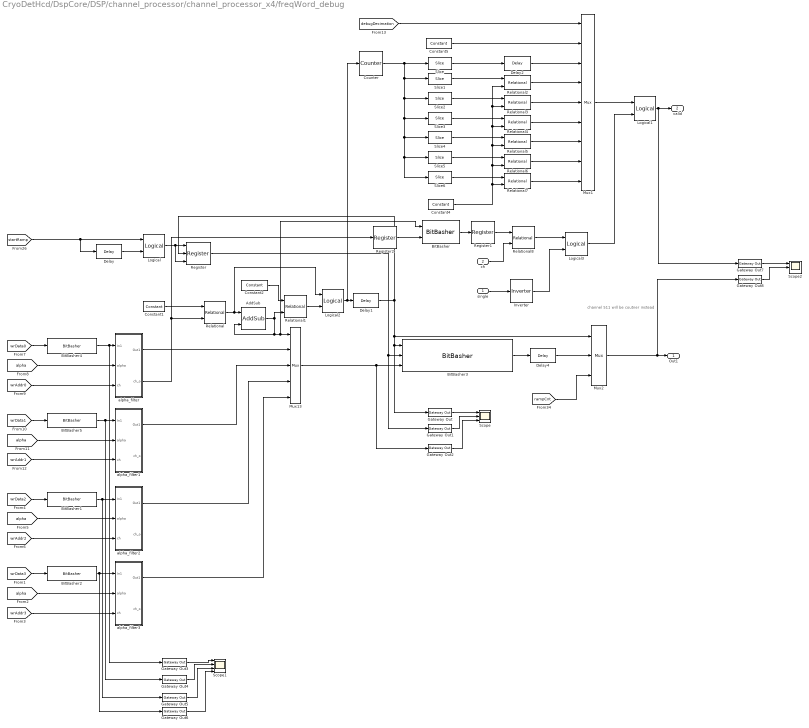
== system CryoDetHcd/DspCore/DSP/channel_processor/channel_processor_x4/freqWord_debug ==
  note: channel 511 will be coutner instead
  single : Inport
  ch : Inport  Port=2
  AddSub : xbsIndex_r4/AddSub  mode=Addition  use_carryin=off  use_carryout=off  en=off  latency=1  precision=User Defined  arith_type=Unsigned  n_bits=2  bin_pt=0  quantization=Truncate  overflow=Wrap  use_behavioral_HDL=off  hw_selection=Fabric  pipelined=off  dbl_ovrd=off  block_type=addsub
  BitBasher : xbsIndex_r4/BitBasher  bitexpr=out = {hi,lo}  display_expr=off  sr_1=out  arith_type1=Unsigned  bin_pt1=0  sr_2=channel_select  arith_type2=Unsigned  bin_pt2=0  sr_3=3  arith_type3=Unsigned  bin_pt3=0  sr_4=4  arith_type4=Unsigned  bin_pt4=0  dbl_ovrd=off  block_type=bitbasher
  BitBasher{1..2,4..5} (4 alike) : xbsIndex_r4/BitBasher  bitexpr=freq = {in[23:0]}  display_expr=on  sr_1=freq  arith_type1=Unsigned  bin_pt1=0  sr_2=2  arith_type2=Unsigned  bin_pt2=0  sr_3=3  arith_type3=Unsigned  bin_pt3=0  sr_4=4  arith_type4=Unsigned  bin_pt4=0  dbl_ovrd=off  block_type=bitbasher
  BitBasher3 : xbsIndex_r4/BitBasher  bitexpr=out = {flux_ramp, ch, 6'b0, freq}  display_expr=on  sr_1=out  arith_type1=Unsigned  bin_pt1=0  sr_2=2  arith_type2=Unsigned  bin_pt2=0  sr_3=3  arith_type3=Unsigned  bin_pt3=0  sr_4=4  arith_type4=Unsigned  bin_pt4=0  dbl_ovrd=off  block_type=bitbasher
  Constant1 : xbsIndex_r4/Constant  const=127  gui_display_data_type=Fixed-point  arith_type=Unsigned  n_bits=7  bin_pt=0  preci_type=Single  exp_width=8  frac_width=24  explicit_period=off  period=1  equ=P=C  opselect=C  inp2=PCIN>>17  opr=+  inp1=P  carry=CIN  dbl_ovrd=off  block_type=constant
  Constant2 : xbsIndex_r4/Constant  const=3  gui_display_data_type=Fixed-point  arith_type=Unsigned  n_bits=2  bin_pt=0  preci_type=Single  exp_width=8  frac_width=24  explicit_period=off  period=1  equ=P=C  opselect=C  inp2=PCIN>>17  opr=+  inp1=P  carry=CIN  dbl_ovrd=off  block_type=constant
  Constant4 : xbsIndex_r4/Constant  const=0  gui_display_data_type=Fixed-point  arith_type=Unsigned  n_bits=1  bin_pt=0  preci_type=Single  exp_width=8  frac_width=24  explicit_period=off  period=1  equ=P=C  opselect=C  inp2=PCIN>>17  opr=+  inp1=P  carry=CIN  dbl_ovrd=off  block_type=constant
  Constant5 : xbsIndex_r4/Constant  const=1  gui_display_data_type=Fixed-point  arith_type=Unsigned  n_bits=1  bin_pt=0  preci_type=Single  exp_width=8  frac_width=24  explicit_period=off  period=1  equ=P=C  opselect=C  inp2=PCIN>>17  opr=+  inp1=P  carry=CIN  dbl_ovrd=off  block_type=constant
  Counter : xbsIndex_r4/Counter  cnt_type=Free Running  cnt_to=Inf  operation=Up  start_count=0  cnt_by_val=1  arith_type=Unsigned  n_bits=7  bin_pt=0  load_pin=off  rst=off  en=on  explicit_period=off  period=2/Fadc  use_behavioral_HDL=off  implementation=Fabric  dbl_ovrd=off  block_type=counter
  Delay{,1..2,4} (4 alike) : xbsIndex_r4/Delay  rst=off  infoeditControl=Selection of Reset will increase slice count due to use of real FFs and instead of SRLs  en=off  latency=1  reg_retiming=off  dbl_ovrd=off  block_type=delay
  Gateway Out{,1..8} (9 alike) : xbsIndex_r4/Gateway Out  inherit_from_input=off  hdl_port=off  rows=1  columns=1  UseAsDAC=off  DACChannel='1'  interface=None  automatic_assignment=on  address_offset=hex2dec('00')  intf_name=''  intf_description=''  timing_constraint=None  locs_specified=off  LOCs={}  io_standard={}  block_type=gatewayout
  Inverter : xbsIndex_r4/Inverter  en=off  latency=0  dbl_ovrd=off  block_type=inv
  Logical : xbsIndex_r4/Logical  logical_function=OR  inputs=2  en=off  latency=1  precision=User Defined  arith_type=Boolean  n_bits=16  bin_pt=0  align_bp=on  dbl_ovrd=off  block_type=logical
  Logical1 : xbsIndex_r4/Logical  logical_function=AND  inputs=2  en=off  latency=0  precision=Full  arith_type=Unsigned  n_bits=16  bin_pt=0  align_bp=on  dbl_ovrd=off  block_type=logical
  Logical2 : xbsIndex_r4/Logical  logical_function=AND  inputs=2  en=off  latency=1  precision=User Defined  arith_type=Boolean  n_bits=16  bin_pt=0  align_bp=on  dbl_ovrd=off  block_type=logical
  Logical3 : xbsIndex_r4/Logical  logical_function=OR  inputs=2  en=off  latency=1  precision=Full  arith_type=Unsigned  n_bits=16  bin_pt=0  align_bp=on  dbl_ovrd=off  block_type=logical
  Mux1 : xbsIndex_r4/Mux  inputs=8  en=off  latency=1  precision=Full  arith_type=Unsigned  n_bits=16  bin_pt=14  quantization=Truncate  overflow=Wrap  dbl_ovrd=off  block_type=mux
  Mux13 : xbsIndex_r4/Mux  inputs=4  en=off  latency=1  precision=Full  arith_type=Unsigned  n_bits=16  bin_pt=14  quantization=Truncate  overflow=Wrap  dbl_ovrd=off  block_type=mux
  Mux2 : xbsIndex_r4/Mux  inputs=2  en=off  latency=1  precision=Full  arith_type=Unsigned  n_bits=16  bin_pt=14  quantization=Truncate  overflow=Wrap  dbl_ovrd=off  block_type=mux
  Register : xbsIndex_r4/Register  init=0  rst=on  en=on  dbl_ovrd=off  block_type=register
  Register1 : xbsIndex_r4/Register  init=0  rst=off  en=off  dbl_ovrd=off  block_type=register
  Register2 : xbsIndex_r4/Register  init=0  rst=off  en=off  dbl_ovrd=off  block_type=register
  Relational{,1..8} (9 alike) : xbsIndex_r4/Relational  mode=a=b  op_type=Ufix  en=off  latency=1  dbl_ovrd=off  block_type=relational
  Scope : Scope  NumInputPorts=3
  Scope1 : Scope  NumInputPorts=4
  Scope2 : Scope  NumInputPorts=3
  Slice : xbsIndex_r4/Slice  nbits=1  boolean_output=off  mode=Lower Bit Location + Width  bit1=0  base1=MSB of Input  bit0=0  base0=LSB of Input  dbl_ovrd=off  block_type=slice
  Slice1 : xbsIndex_r4/Slice  nbits=2  boolean_output=off  mode=Lower Bit Location + Width  bit1=0  base1=MSB of Input  bit0=0  base0=LSB of Input  dbl_ovrd=off  block_type=slice
  Slice2 : xbsIndex_r4/Slice  nbits=3  boolean_output=off  mode=Lower Bit Location + Width  bit1=0  base1=MSB of Input  bit0=0  base0=LSB of Input  dbl_ovrd=off  block_type=slice
  Slice3 : xbsIndex_r4/Slice  nbits=4  boolean_output=off  mode=Lower Bit Location + Width  bit1=0  base1=MSB of Input  bit0=0  base0=LSB of Input  dbl_ovrd=off  block_type=slice
  Slice4 : xbsIndex_r4/Slice  nbits=5  boolean_output=off  mode=Lower Bit Location + Width  bit1=0  base1=MSB of Input  bit0=0  base0=LSB of Input  dbl_ovrd=off  block_type=slice
  Slice5 : xbsIndex_r4/Slice  nbits=6  boolean_output=off  mode=Lower Bit Location + Width  bit1=0  base1=MSB of Input  bit0=0  base0=LSB of Input  dbl_ovrd=off  block_type=slice
  Slice6 : xbsIndex_r4/Slice  nbits=7  boolean_output=off  mode=Lower Bit Location + Width  bit1=0  base1=MSB of Input  bit0=0  base0=LSB of Input  dbl_ovrd=off  block_type=slice
  alpha_filter : Subsystem
  alpha_filter1 : Subsystem
  alpha_filter2 : Subsystem
  alpha_filter3 : Subsystem
  Out1 : Outport
  valid : Outport  Port=2
  wires:
  [wrData1] -> BitBasher5/1
  [alpha] -> alpha_filter1/2(alpha)
  [wrAddr0] -> alpha_filter/3(ch)
  [wrAddr1] -> alpha_filter1/3(ch)
  BitBasher5/1 -> Gateway Out4/1, alpha_filter1/1(In1)
  [alpha] -> alpha_filter/2(alpha)
  [wrData0] -> BitBasher4/1
  BitBasher4/1 -> Gateway Out3/1, alpha_filter/1(In1)
  [wrData3] -> BitBasher2/1
  [alpha] -> alpha_filter3/2(alpha)
  [wrAddr2] -> alpha_filter2/3(ch)
  [wrAddr3] -> alpha_filter3/3(ch)
  BitBasher2/1 -> Gateway Out6/1, alpha_filter3/1(In1)
  [alpha] -> alpha_filter2/2(alpha)
  [wrData2] -> BitBasher1/1
  BitBasher1/1 -> Gateway Out5/1, alpha_filter2/1(In1)
  alpha_filter/1(Out1) -> Mux13/2
  alpha_filter1/1(Out1) -> Mux13/3
  alpha_filter2/1(Out1) -> Mux13/4
  alpha_filter3/1(Out1) -> Mux13/5
  Delay/1 -> Logical/2
  [startRamp] -> Delay/1, Logical/1
  Logical/1 -> Register/3, Register/1
  alpha_filter/2(ch_o) -> Register2/1, Relational/2
  Constant1/1 -> Relational/1
  Constant2/1 -> Relational1/1
  BitBasher3/1 -> Delay4/1
  Mux13/1 -> Gateway Out2/1, BitBasher3/3
  Relational1/1 -> Logical2/2
  Register/1 -> Gateway Out1/1, BitBasher3/2
  Relational/1 -> Logical2/1, AddSub/1
  AddSub/1 -> AddSub/2, BitBasher/1, Mux13/1, Relational1/2
  Gateway Out/1 -> Scope/1
  Gateway Out1/1 -> Scope/2
  Gateway Out2/1 -> Scope/3
  Gateway Out3/1 -> Scope1/1
  Gateway Out4/1 -> Scope1/2
  Gateway Out5/1 -> Scope1/3
  Gateway Out6/1 -> Scope1/4
  Delay1/1 -> Register/2, Mux2/1, Gateway Out/1, BitBasher3/1
  Counter/1 -> Slice3/1, Slice4/1, Slice5/1, Slice6/1, Slice2/1, Slice1/1, Slice/1
  Logical2/1 -> Counter/1, Delay1/1
  Slice1/1 -> Relational2/1
  Slice2/1 -> Relational3/1
  Constant4/1 -> Relational2/2, Relational3/2, Relational4/2, Relational5/2, Relational6/2, Relational7/2
  Relational7/1 -> Mux1/9
  Relational6/1 -> Mux1/8
  Relational5/1 -> Mux1/7
  Relational4/1 -> Mux1/6
  Relational3/1 -> Mux1/5
  Relational2/1 -> Mux1/4
  Delay2/1 -> Mux1/3
  Slice/1 -> Delay2/1
  Slice3/1 -> Relational4/1
  Slice4/1 -> Relational5/1
  Slice5/1 -> Relational6/1
  Slice6/1 -> Relational7/1
  Constant5/1 -> Mux1/2
  Delay4/1 -> Mux2/2
  Mux2/1 -> Gateway Out8/1, Out1/1
  [rampCnt] -> Mux2/3
  [debugDecimation] -> Mux1/1
  BitBasher/1 -> Register1/1
  Register2/1 -> BitBasher/2
  Mux1/1 -> Logical1/1
  Logical1/1 -> Gateway Out7/1, valid/1
  Register1/1 -> Relational8/1
  Relational8/1 -> Logical3/1
  Logical3/1 -> Logical1/2
  ch/1 -> Relational8/2
  single/1 -> Inverter/1
  Inverter/1 -> Logical3/2
  Gateway Out7/1 -> Scope2/1
  Gateway Out8/1 -> Scope2/2
